simulink model "Robertson_problem"  (R2012b)
settings: Solver=ode23tb  StartTime=0  StopTime=4*1e6  RelTol=1e-6
settings Model: Creator=David  LastModifiedBy=David
settings DataIOCC: SignalLoggingSaveFormat=ModelDataLogs
settings DebuggingCC: FcnCallInpInsideContextMsg=UseLocalSettings
settings RTWCC: TargetLang=C++
settings GRTTargetCC: CombineOutputUpdateFcns=off  GRTInterface=on

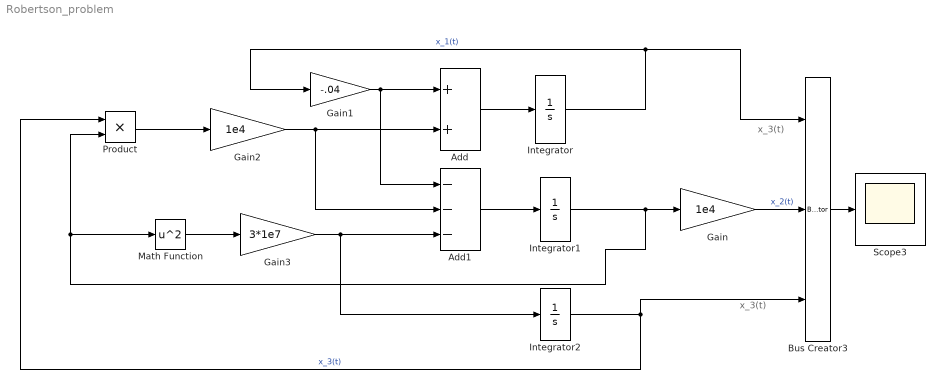
== system Robertson_problem ==
  note: x_3(t)
  note: x_3(t)
  Add : Sum
  Add1 : Sum  Inputs=---
  Bus Creator3 : BusCreator  Inputs=3
  Gain : Gain  Gain=1e4
  Gain1 : Gain  Gain=-.04
  Gain2 : Gain  Gain=1e4
  Gain3 : Gain  Gain=3*1e7
  Integrator : Integrator  InitialCondition=1
  Integrator1 : Integrator
  Integrator2 : Integrator
  Math Function : Math  Operator=square  SaturateOnIntegerOverflow=on
  Product : Product  RndMeth=Zero
  Scope3 : Scope
      settings: ShowLegends=on  SaveName=ScopeData3  SampleInput=on
  wires:
  Integrator/1 -> Bus Creator3/1, Gain1/1  "x_1(t)"
  Add/1 -> Integrator/1
  Integrator1/1 -> Math Function/1, Product/2, Gain/1
  Integrator2/1 -> Bus Creator3/3, Product/1  "x_3(t)"
  Add1/1 -> Integrator1/1
  Gain/1 -> Bus Creator3/2  "x_2(t)"
  Bus Creator3/1 -> Scope3/1
  Gain1/1 -> Add/1, Add1/1
  Gain2/1 -> Add1/2, Add/2
  Product/1 -> Gain2/1
  Math Function/1 -> Gain3/1
  Gain3/1 -> Add1/3, Integrator2/1
